simulink model "mqam_model_inclass"  (R2021b)
settings: Solver=VariableStepAuto  StartTime=0.0  StopTime=10.0  RelTol=1e-3
values from neighbouring files (symbols this model uses):
  Tb = 1/Rb    [question1a.m]    (also in question1b.m)
libraries: commutil2 x2, commdigbbndam3 x2, commchan3 x1, commrandsrc3 x1, commsink2 x1
settings Model: Creator=enes_  LastModifiedBy=enes_

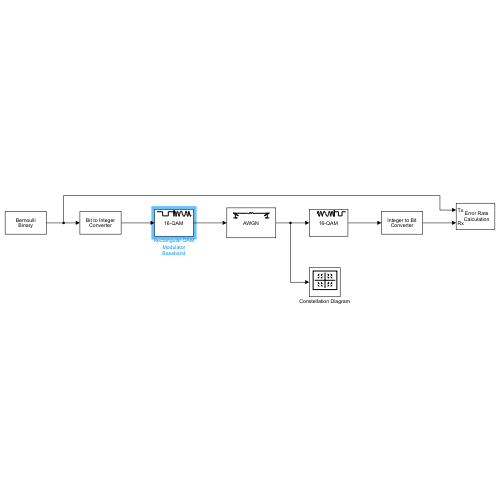
[thumbnail: Simulink's stored preview of the top-level diagram]
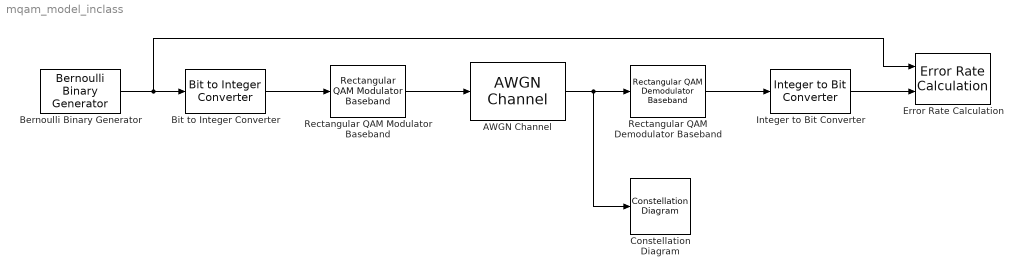
== system mqam_model_inclass ==
  AWGN Channel : commchan3/AWGN Channel  InputProcessing=Columns as channels (frame based)  seed=67  noiseMode="Signal to noise ratio  (Eb/No)"  EbNodB=EbN0dB  EsNodB=10  SNRdB=10  bitsPerSym=L  Ps=1  Tsym=Ts  variance=1
  Bernoulli Binary Generator : commrandsrc3/Bernoulli Binary Generator  ProbabilityOfZero=0.5  SeedSource=Auto  Seed=0  SampleTime=Tb  SamplesPerFrame=3600  OutputDataType=double  SimulateUsing=Interpreted execution
  Bit to Integer Converter : commutil2/Bit to Integer Converter  nbits=L  bitOrder=MSB first  signedOutputValues=Unsigned  outDtype=Inherit via internal rule  outDtypeSigned=Inherit via internal rule
  Constellation Diagram : ConstellationDiagram
  Error Rate Calculation : commsink2/Error Rate Calculation  N=0  st_delay=0  cp_mode=Entire frame  subframe=[]  PMode=Workspace  WsName=ErrorVec  RsMode2=off  stop=off  numErr=100  maxBits=1e6
  Integer to Bit Converter : commutil2/Integer to Bit Converter  nbits=L  signedInputValues=Unsigned  bitOrder=MSB first  outDtype=Inherit via internal rule
  Rectangular QAM Demodulator Baseband : commdigbbndam3/Rectangular QAM Demodulator Baseband  M=M  OutType=Integer  DecType=Hard decision  VarSource=Dialog  Variance=1  Dec=Gray  Mapping=[0:15]  PowType=Average Power  MinDist=2  AvgPow=1  PeakPow=1  Ph=0  outDtype1=Inherit via internal rule  outDtype2=Inherit via internal rule  derotateFactorWordLen=16  derotateFactorDataTypeStr=Inherit: Same word length as input  derotateFactorLastDataTypeStr=Inherit: Same word length as input  denormFactorWordLen=16  denormFactorDataTypeStr=Inherit: Same word length as input  denormFactorLastDataTypeStr=Inherit: Same word length as input  prodOutWordLen=32  prodOutOverflowMode=Wrap  prodOutRoundingMode=Floor  prodOutOvFlMode=off  prodOutOvFlModeLastStrValue=off  sumWordLen=32
  Rectangular QAM Modulator Baseband : commdigbbndam3/Rectangular QAM Modulator Baseband  M=M  InType=Integer  Enc=Gray  Mapping=[0:15]  PowType=Average Power  MinDist=2  AvgPow=1  PeakPow=1  Ph=0  outDtype=double  outWordLen=16  outUDDataType=sfix(16)  outFracLenMode=Best precision  outFracLen=15  outDataTypeStr=double  outLastDataTypeStr=double
  wires:
  Bernoulli Binary Generator/1 -> Error Rate Calculation/1, Bit to Integer Converter/1
  Rectangular QAM Modulator Baseband/1 -> AWGN Channel/1
  AWGN Channel/1 -> Rectangular QAM Demodulator Baseband/1, Constellation Diagram/1
  Rectangular QAM Demodulator Baseband/1 -> Integer to Bit Converter/1
  Integer to Bit Converter/1 -> Error Rate Calculation/2
  Bit to Integer Converter/1 -> Rectangular QAM Modulator Baseband/1
